simulink model "RK4_simulink"  (R2023b)
settings: Solver=ode4  StartTime=t0  StopTime=tf  FixedStep=dt  RelTol=1e-3
settings Model: Creator=Ahmed Raamadan  LastModifiedBy=Ahmed Raamadan

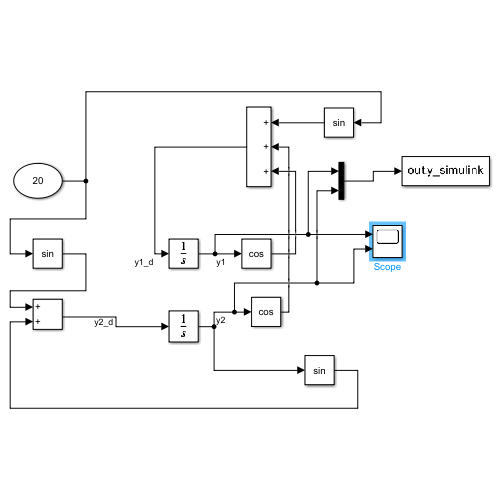
[thumbnail: Simulink's stored preview of the top-level diagram]
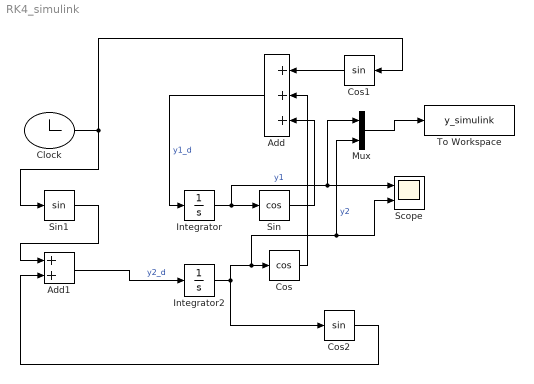
== system RK4_simulink ==
  Add : Sum  Inputs=+++
  Add1 : Sum
  Clock : Clock
  Cos : Trigonometry  Operator=cos
  Cos1 : Trigonometry
  Cos2 : Trigonometry
  Integrator : Integrator  InitialCondition=2
  Integrator2 : Integrator  InitialCondition=1
  Mux : Mux  Inputs=2
  Scope : Scope  NumInputPorts=2
  Sin : Trigonometry  Operator=cos
  Sin1 : Trigonometry
  To Workspace : ToWorkspace  VariableName=y_simulink  SampleTime=-1
  wires:
  Integrator2/1 -> Cos2/1, Mux/2, Scope/2, Cos/1  "y2"
  Clock/1 -> Sin1/1, Cos1/1
  Cos1/1 -> Add/1
  Mux/1 -> To Workspace/1
  Sin1/1 -> Add1/1
  Cos/1 -> Add/2
  Add1/1 -> Integrator2/1  "y2_d"
  Integrator/1 -> Mux/1, Scope/1, Sin/1  "y1"
  Add/1 -> Integrator/1  "y1_d"
  Sin/1 -> Add/3
  Cos2/1 -> Add1/2
